simulink model "SingleCylinderSparkIgnitionEngine_apple2"  (R2024b)
settings: Solver=VariableStepAuto  StartTime=0.0  StopTime=40  RelTol=1e-3
libraries: nesl_utility x10, fl_lib x8, sdl_lib x1
CloseFcn:
  | try, close(h1_SingleCylinderSparkIgnitionEngine), end
  | clear h1_SingleCylinderSparkIgnitionEngine
  | 
  | clear simlog_SingleCylinderSparkIgnitionEngine
  | clear logsout_SingleCylinderSparkIgnitionEngine
settings Model: PacingRate=0.040000  Creator=The MathWorks, Inc.  LastModifiedBy=jc790999
settings SolverCC: MaxZcPerStep=1
settings DataIOCC: SaveOutput=off  DSMLogging=off
settings ModelReferenceCC: EnableRefExpFcnMdlSchedulingChecks=on
settings RTWCC: GPUComputeCapability=3.5  DLArmComputeVersion=19.05
settings SimscapeCC: SimscapeLogType=all  SimscapeLogSimulationStatistics=on  SimscapeLogLimitData=off

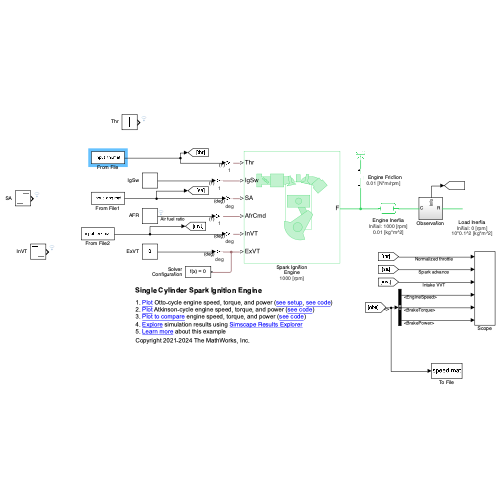
[thumbnail: Simulink's stored preview of the top-level diagram]
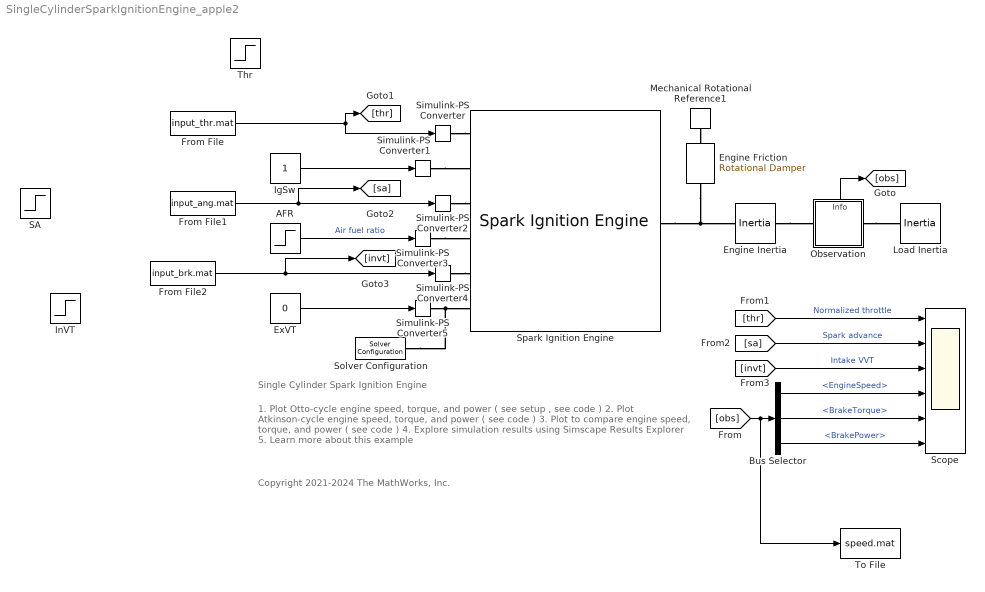
== system SingleCylinderSparkIgnitionEngine_apple2 ==
  note: Single Cylinder Spark Ignition Engine
  note: Copyright 2021-2024 The MathWorks, Inc.
  note: 1. Plot Otto-cycle engine speed, torque, and power ( see setup , see code )
      | 2. Plot Atkinson-cycle engine speed, torque, and power ( see code )
      | 3. Plot to compare engine speed, torque, and power ( see code )
      | 4. Explore simulation results using Simscape Results Explorer
      | 5. Learn more about this example
  AFR : Step  Time=1.5  Before=13.0  After=14.6  SampleTime=0
  Bus Selector : BusSelector  OutputSignals=EngineSpeed,BrakeTorque,BrakePower
  Engine Friction : fl_lib/Mechanical/Rotational Elements/Rotational Damper  D=0.01 N*m/rpm  w_specify=off  w_priority=None  w=0 rad/s  w_nominal_specify=off  w_nominal_value=1  w_nominal_unit=rad/s  t_specify=off  t_priority=None  t=0 N*m  t_nominal_specify=off  t_nominal_value=1  t_nominal_unit=N*m
      settings: AttributesFormatString=%<D> [%<D_unit>]
  Engine Inertia : fl_lib/Mechanical/Rotational Elements/Inertia  inertia=0.01 kg*m^2  num_ports=foundation.enum.numPorts2.two  w_specify=on  w_priority=High  w=1000 rpm  w_nominal_specify=off  w_nominal_value=1  w_nominal_unit=rad/s  t_specify=off  t_priority=None  t=0 N*m  t_nominal_specify=off  t_nominal_value=1  t_nominal_unit=N*m
      settings: InternalSimscapePortConfiguration="{\"Bottom\":[],\"Left\":[{\"id\":\"I\",\"label\":\"\",\"type\":\"foundation.mechanical.rotational.rotational\"}],\"Right\":[{\"id\":\"J\",\"label\":\"\",\"type\":\"foundation.mechanical.rotational.rotational\"}],\"Top\":[]}"
      settings: AttributesFormatString=|
      | Initial: %<w> [%<w_unit>]
      | %<inertia> [%<inertia_unit>]
  ExVT : Constant  Value=0
  From File : FromFile  FileName=input_thr.mat  OutDataTypeStr=double  SampleTime=0
  From File1 : FromFile  FileName=input_ang.mat  OutDataTypeStr=double  SampleTime=0
  From File2 : FromFile  FileName=input_brk.mat  OutDataTypeStr=double  SampleTime=0
  IgSw : Constant
  InVT : Step  Time=3  Before=30  After=0  SampleTime=0
  Load Inertia : fl_lib/Mechanical/Rotational Elements/Inertia  inertia=10*0.1^2 kg*m^2  num_ports=foundation.enum.numPorts2.one  w_specify=on  w_priority=None  w=0 rpm  w_nominal_specify=off  w_nominal_value=1  w_nominal_unit=rad/s  t_specify=off  t_priority=None  t=0 N*m  t_nominal_specify=off  t_nominal_value=1  t_nominal_unit=N*m
      settings: AttributesFormatString=|
      | Initial: %<w> [%<w_unit>]
      | %<inertia> [%<inertia_unit>]
  Mechanical Rotational Reference1 : fl_lib/Mechanical/Rotational Elements/Mechanical Rotational Reference
  Observation : Subsystem
      settings: PortSchema="{\"entries\":[{\"content\":{\"sides\":[{\"content\":{\"connectorIds\":[\"LConn1\"]},\"type\":\"ConnectorPlacement.EquallySpacedRectSide\",\"uuid\":\"410be9a6-c4e5-432d-8066-24e0f4965a53\"},{\"content\":{\"connectorIds\":[\"RConn1\"],\"side\":\"RIGHT\"},\"type\":\"ConnectorPlacement.EquallySpacedRectSide\",\"uuid\":\"7b59f0c0-a218-4635-982c-3ab19ae33344\"},{\"content\":{\"connectorIds\":[\"Out1\"],\"side\":\"TOP\"},\"type\":\"ConnectorPlacement.EquallySpacedRectSide\",\"uuid\":\"569b4327-99bc-47a9-a8b7-c1caa6dee46d\"}]},\"type\":\"ConnectorPlacement.EquallySpacedConnector\",\"uuid\":\"611a8619-a64a-4be7-a61a-aa8fabb87e61\"}],\"packageUris\":[\"http://schema.mathworks.com/mf0/Connector/R2020b\"],\"version\":\"1.0\"}"
  SA : Step  Time=2  Before=10  After=30  SampleTime=0
  Scope : Scope  NumInputPorts=6
  Simulink-PS Converter : nesl_utility/Simulink-PS Converter  PhysicalDomain=network_engine_domain  SubClassName=ps_input  LeftPortType=input  RightPortType=output  PseudoPeriodic=off  Frequencies=[]  NoiseDistribution=none  NoiseParameters=[]  Unit=1  AffineConversion=off  FilteringAndDerivatives=provide  SimscapeFilterOrder=1  InputFilterTimeConstant=0.001  UdotUserProvided=0
  Simulink-PS Converter1 : nesl_utility/Simulink-PS Converter  PhysicalDomain=network_engine_domain  SubClassName=ps_input  LeftPortType=input  RightPortType=output  PseudoPeriodic=off  Frequencies=[]  NoiseDistribution=none  NoiseParameters=[]  Unit=1  AffineConversion=off  FilteringAndDerivatives=provide  SimscapeFilterOrder=1  InputFilterTimeConstant=0.001  UdotUserProvided=0
  Simulink-PS Converter2 : nesl_utility/Simulink-PS Converter  PhysicalDomain=network_engine_domain  SubClassName=ps_input  LeftPortType=input  RightPortType=output  PseudoPeriodic=off  Frequencies=[]  NoiseDistribution=none  NoiseParameters=[]  Unit=deg  AffineConversion=off  FilteringAndDerivatives=provide  SimscapeFilterOrder=1  InputFilterTimeConstant=0.001  UdotUserProvided=0
  Simulink-PS Converter3 : nesl_utility/Simulink-PS Converter  PhysicalDomain=network_engine_domain  SubClassName=ps_input  LeftPortType=input  RightPortType=output  PseudoPeriodic=off  Frequencies=[]  NoiseDistribution=none  NoiseParameters=[]  Unit=1  AffineConversion=off  FilteringAndDerivatives=provide  SimscapeFilterOrder=1  InputFilterTimeConstant=0.001  UdotUserProvided=0
  Simulink-PS Converter4 : nesl_utility/Simulink-PS Converter  PhysicalDomain=network_engine_domain  SubClassName=ps_input  LeftPortType=input  RightPortType=output  PseudoPeriodic=off  Frequencies=[]  NoiseDistribution=none  NoiseParameters=[]  Unit=deg  AffineConversion=off  FilteringAndDerivatives=provide  SimscapeFilterOrder=1  InputFilterTimeConstant=0.001  UdotUserProvided=0
  Simulink-PS Converter5 : nesl_utility/Simulink-PS Converter  PhysicalDomain=network_engine_domain  SubClassName=ps_input  LeftPortType=input  RightPortType=output  PseudoPeriodic=off  Frequencies=[]  NoiseDistribution=none  NoiseParameters=[]  Unit=deg  AffineConversion=off  FilteringAndDerivatives=provide  SimscapeFilterOrder=1  InputFilterTimeConstant=0.001  UdotUserProvided=0
  Solver Configuration : nesl_utility/Solver Configuration  PhysicalDomain=network_engine_domain  SubClassName=solver  LeftPortType=input  RightPortType=generic  Tones=[]  Harmonics=[]  SimulateNoise=off  Profile=off  UseLocalSampling=off  EnableSwitchedLinearOptims=on  FrequencyDomain=off  UseCCode=off  RelTol=0.001  AbsTol=0.001  MinStep=1e-09  ToWorkspace=off  RevertToSquareIcSolve=off  NumHomotopyIterations=100  PhasorMode=off  PhasorModeNumHarmonics=1  ConsistencySolver=NEWTON_XTOL_AFTER_FTOL  IndexReductionMethod=DerivativeReplacement  DoDC=off  ResidualTolerance=1e-09  ConsistencyTolSource=GLOBAL  ConsistencyAbsTol=0.001  ConsistencyRelTol=0.001  ConsistencyTolFactor=0.001  UseLocalSolver=off  LocalSolverChoice=NE_BACKWARD_EULER_ADVANCER  ResolveIndetEquations=on  FunctionEvalNumThread=1  LocalSolverSampleTime=0.001  DoFixedCost=off  MaxNonlinIter=3  MaxModeIter=2  ComputeImpulses=off  ImpulseIterations=2  LinearAlgebra=auto  LinearAlgebraNumThread=0  EquationFormulation=NE_TIME_EF  DelaysMemoryBudget=1024  AutomaticFiltering=on  FilteringTimeConstant=0.001  PartitionStorageMethod=AS_NEEDED  PartitionMemoryBudget=1024  PartitionMethod=ROBUST  MultibodyUseLocalSolver=off  MultibodyLocalSolverChoice=ODE1  MultibodyLocalSolverSampleTime=0.001
  Spark Ignition Engine : sdl_lib/Engines & Motors/Spark Ignition Engine  numCyls=sdl.enum.engineNumCylinders.One  twoCylSADiff=270 deg  L4FiringOrder=sdl.enum.engineFiringOrderFourCylinders.L4_1342  bore=72 mm  stroke=61 mm  conrod=97 mm  CR=13  P_amb=101.325 kPa  T_amb=298.15 K  rho_air=1.225 mg/cm^3  R_air=288.1965 J/(K*kg)  UseAirIntake=simscape.enum.onoff.on  c_thr=0.05 s  thr_rest=3 deg  D_plate=5 cm  S_leak=1 cm^2  V_im=500 cm^3  Cd_in=0.9  IVO_0=-10 deg  IVC_0=100 deg  EVO_0=30 deg  EVC_0=5 deg  UseInVVT=simscape.enum.onoff.on  UseExVVT=simscape.enum.onoff.on  q_LHV=44.3 MJ/kg  InputAFR=simscape.enum.onoff.on  AFR_const=14.6  InputInjPw=simscape.enum.onoff.off  Sinj=6.5 mg/ms  SparkInputType=sdl.enum.engineSparkInputType.Angle  SA_const=20 deg  comb_bd=50 deg  dt_Pcyl_slow_decay=60 s  dt_Tcyl_slow_decay=600 s  dt_exh_decay=5 ms  InputBackPressure=simscape.enum.onoff.off  dP_exh=50 kPa  dw_exh=6000 rpm  UseExhaustThermal=simscape.enum.onoff.on  S_exh=1 m^2  M_exh=5 kg  C_exh=100 J/(K*kg)  k_gas=10 s  h_convection=100 W/(K*m^2)  k_radiation=0.3  SB=5.7e-8 W/(K^4*m^2)  Pim_0=101.325 kPa  ca0=0 deg  w0=1000 rpm  EngSpdSimLimit=10000 rpm  OutputTorqueAvr=simscape.enum.onoff.off  OutputSpeedAvr=simscape.enum.onoff.off  OutputCrkpos=simscape.enum.onoff.off  OutputPim=simscape.enum.onoff.off  OutputAirMassFlow=simscape.enum.onoff.off  OutputFuelMassFlow=simscape.enum.onoff.off  OutputAFR=simscape.enum.onoff.off  OutputVcyl=simscape.enum.onoff.off  OutputPcyl=simscape.enum.onoff.off  OutputTcyl=simscape.enum.onoff.off  OutputTexh=simscape.enum.onoff.off
      settings: AttributesFormatString=%<w0> [%<w0_unit>]  InternalSimscapePortConfiguration="{\"Bottom\":[],\"Left\":[{\"id\":\"thr_cmd\",\"label\":\"Thr\",\"type\":\"input\"},{\"id\":\"IGSW\",\"label\":\"IgSw\",\"type\":\"input\"},{\"id\":\"sa\",\"label\":\"SA\",\"type\":\"input\"},{\"id\":\"afr_in\",\"label\":\"AfrCmd\",\"type\":\"input\"},{\"id\":\"dIV\",\"label\":\"InVT\",\"type\":\"input\"},{\"id\":\"dEV\",\"label\":\"ExVT\",\"type\":\"input\"}],\"Right\":[{\"id\":\"F\",\"label\":\"F\",\"type\":\"foundation.mechanical.rotational.rotational\"}],\"Top\":[]}"
  Thr : Step  Before=0.2  SampleTime=0
  To File : ToFile  Filename=speed.mat  SaveFormat=Timeseries
  wires:
  IgSw/1 -> Simulink-PS Converter1/1
  AFR/1 -> Simulink-PS Converter3/1  "Air fuel ratio"
  ExVT/1 -> Simulink-PS Converter5/1
  Observation/1(Info) -> [obs]
  [thr] -> Scope/1  "Normalized throttle"
  [sa] -> Scope/2  "Spark advance"
  [invt] -> Scope/3  "Intake VVT"
  Bus Selector/1 -> Scope/4  "<EngineSpeed>"
  Bus Selector/2 -> Scope/5  "<BrakeTorque>"
  Bus Selector/3 -> Scope/6  "<BrakePower>"
  From File/1 -> [thr], Simulink-PS Converter/1
  From File1/1 -> [sa], Simulink-PS Converter2/1
  From File2/1 -> Simulink-PS Converter4/1, [invt]
  [obs] -> To File/1, Bus Selector/1
  connections:
  Simulink-PS Converter/RConn1 -- Spark Ignition Engine/LConn1
  Simulink-PS Converter1/RConn1 -- Spark Ignition Engine/LConn2
  Simulink-PS Converter2/RConn1 -- Spark Ignition Engine/LConn3
  Simulink-PS Converter3/RConn1 -- Spark Ignition Engine/LConn4
  Simulink-PS Converter4/RConn1 -- Spark Ignition Engine/LConn5
  Simulink-PS Converter5/RConn1 -- Solver Configuration/RConn1 -- Spark Ignition Engine/LConn6
  Mechanical Rotational Reference1/LConn1 -- Engine Friction/RConn1
  Observation/RConn1 -- Load Inertia/LConn1
  Spark Ignition Engine/RConn1 -- Engine Friction/LConn1 -- Engine Inertia/RConn1
  Engine Inertia/LConn1 -- Observation/LConn1

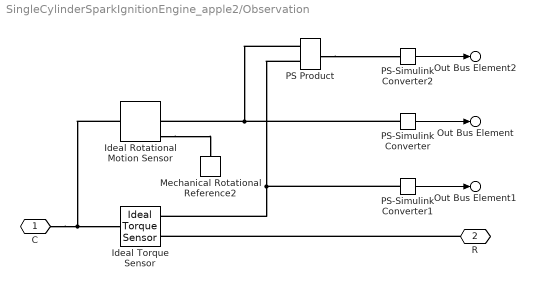
== system SingleCylinderSparkIgnitionEngine_apple2/Observation ==
  Ideal Rotational Motion Sensor : fl_lib/Mechanical/Mechanical Sensors/Ideal Rotational Motion Sensor  reference=foundation.enum.MeasurementReference.difference  acceleration_port=false  velocity_port=true  position_port=true  wrap_angle=simscape.enum.onoff.off  offset=0 rad
  Ideal Torque Sensor : fl_lib/Mechanical/Mechanical Sensors/Ideal Torque Sensor
  Mechanical Rotational Reference2 : fl_lib/Mechanical/Rotational Elements/Mechanical Rotational Reference
  PS Product : fl_lib/Physical Signals/Functions/PS Product
  PS-Simulink Converter : nesl_utility/PS-Simulink Converter  PhysicalDomain=network_engine_domain  SubClassName=ps_output  LeftPortType=input  RightPortType=output  PseudoPeriodic=off  Frequencies=[]  VectorFormat=inherit  Unit=rpm  AffineConversion=off
  PS-Simulink Converter1 : nesl_utility/PS-Simulink Converter  PhysicalDomain=network_engine_domain  SubClassName=ps_output  LeftPortType=input  RightPortType=output  PseudoPeriodic=off  Frequencies=[]  VectorFormat=inherit  Unit=N*m  AffineConversion=off
  PS-Simulink Converter2 : nesl_utility/PS-Simulink Converter  PhysicalDomain=network_engine_domain  SubClassName=ps_output  LeftPortType=input  RightPortType=output  PseudoPeriodic=off  Frequencies=[]  VectorFormat=inherit  Unit=kW  AffineConversion=off
  C : PMIOPort  Side=Left
  R : PMIOPort  Port=2  Side=Right
  Out Bus Element : Outport  PortName=Info  Element=EngineSpeed
      settings: AttributesFormatString=%<Unit>
  Out Bus Element1 : Outport  PortName=Info  Element=BrakeTorque
      settings: AttributesFormatString=%<Unit>
  Out Bus Element2 : Outport  PortName=Info  Element=BrakePower
      settings: AttributesFormatString=%<Unit>
  wires:
  PS-Simulink Converter/1 -> Out Bus Element/1
  PS-Simulink Converter1/1 -> Out Bus Element1/1
  PS-Simulink Converter2/1 -> Out Bus Element2/1
  connections:
  Ideal Rotational Motion Sensor/RConn1 -- Mechanical Rotational Reference2/LConn1
  Ideal Rotational Motion Sensor/LConn1 -- C/RConn1 -- Ideal Torque Sensor/LConn1
  PS-Simulink Converter/LConn1 -- PS Product/LConn1 -- Ideal Rotational Motion Sensor/RConn2
  PS-Simulink Converter1/LConn1 -- PS Product/LConn2 -- Ideal Torque Sensor/RConn2
  R/RConn1 -- Ideal Torque Sensor/RConn1
  PS Product/RConn1 -- PS-Simulink Converter2/LConn1
